simulink library "mRefLib"  (R2024a)
settings: Solver=VariableStepAuto  StartTime=0.0  StopTime=10.0  RelTol=1e-3
settings Model: Creator=uditpant  LastModifiedBy=uditpant

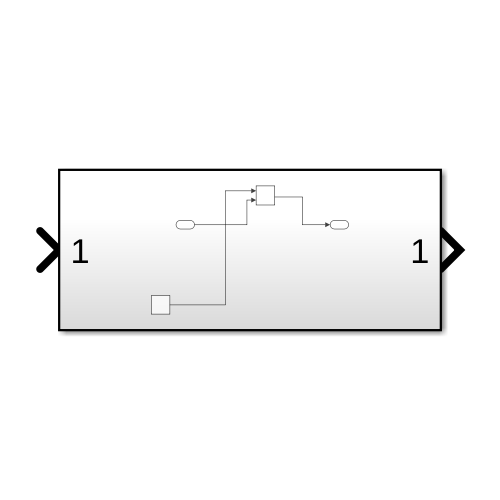
[thumbnail: Simulink's stored preview of the top-level diagram]
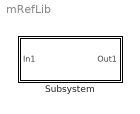
== system mRefLib ==
  Subsystem : Subsystem

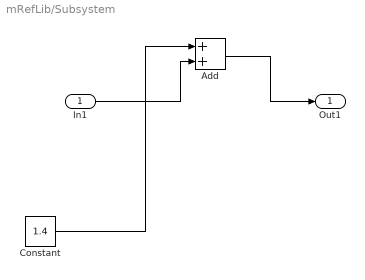
== system mRefLib/Subsystem ==
  In1 : Inport
  Add : Sum
  Constant : Constant  Value=1.4
  Out1 : Outport
  wires:
  In1/1 -> Add/2
  Constant/1 -> Add/1
  Add/1 -> Out1/1
